simulink model "Simulation"  (R2021b)
settings: Solver=FixedStepAuto  StartTime=0.0  StopTime=30  FixedStep=Ts  RelTol=1e-3
InitFcn:
  | Tf = 200;
  | Ts = 0.01;
  | T = 0:Ts:Tf;
  | rolla = T';
  | omegaa=T';
  | omegax =T';
  | %%
  | 
  | load('A');
  | A = A(2001:2000+length(T),:);
  | rolla(:,2) = A(:,2)-0.0661;
  | omegaa(:,2) = A(:,1);
  | omegax(:,2) = A(:,3);
  | %%
  | l1 =10;
  | initial_vector_error = ones(1,l1)*0.001;
  | initial_vector_error(1) = 0.001;
undefined symbols (not defined in the file or in its folder): X, Y, Z
libraries: nesl_utility x23, sm_lib x15, simulink x3
(part 2 of 2)

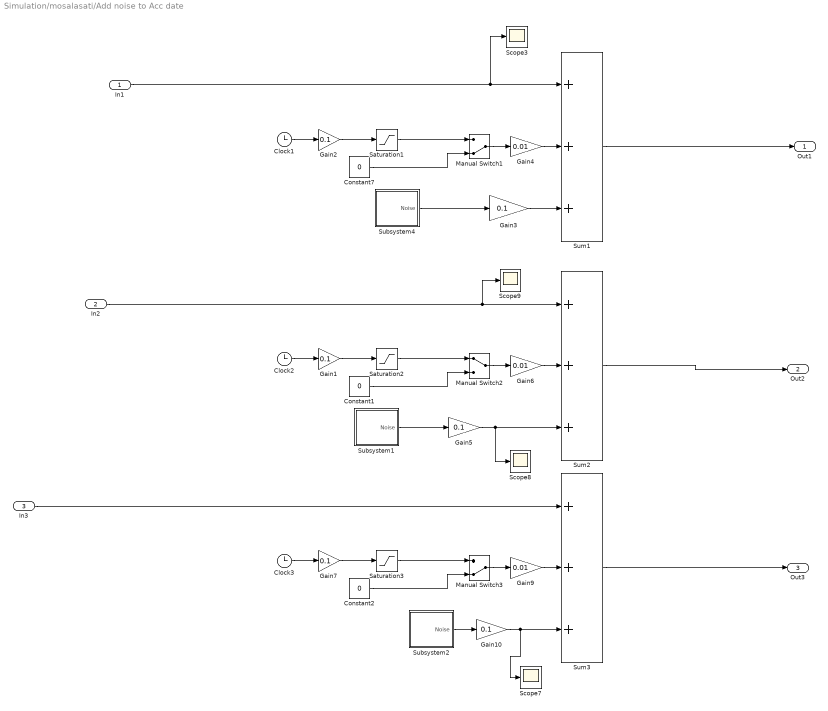
== system Simulation/mosalasati/Add noise to Acc date ==
  In1 : Inport
  In2 : Inport  Port=2
  In3 : Inport  Port=3
  Clock1 : Clock
  Clock2 : Clock
  Clock3 : Clock
  Constant1 : Constant  Value=0
  Constant2 : Constant  Value=0
  Constant7 : Constant  Value=0
  Gain{1..3,5,7,10} (6 alike) : Gain  Gain=0.1
  Gain4 : Gain  Gain=0.01
  Gain6 : Gain  Gain=0.01
  Gain9 : Gain  Gain=0.01
  Manual Switch1 : ManualSwitch  CurrentSetting=0
  Manual Switch2 : ManualSwitch
  Manual Switch3 : ManualSwitch  CurrentSetting=0
  Saturation1 : Saturate  UpperLimit=5
  Saturation2 : Saturate  UpperLimit=5
  Saturation3 : Saturate  UpperLimit=5
  Scope{3,7..9} (4 alike) : Scope
  Subsystem1 : Subsystem
  Subsystem2 : Subsystem
  Subsystem4 : Subsystem
  Sum1 : Sum  Inputs=+++
  Sum2 : Sum  Inputs=+++
  Sum3 : Sum  Inputs=+++
  Out1 : Outport  VectorParamsAs1DForOutWhenUnconnected=off
  Out2 : Outport  Port=2  VectorParamsAs1DForOutWhenUnconnected=off
  Out3 : Outport  Port=3  VectorParamsAs1DForOutWhenUnconnected=off
  wires:
  In2/1 -> Sum2/1, Scope9/1
  Saturation2/1 -> Manual Switch2/1
  Constant1/1 -> Manual Switch2/2
  Gain6/1 -> Sum2/2
  Manual Switch1/1 -> Gain4/1
  Manual Switch2/1 -> Gain6/1
  Sum1/1 -> Out1/1
  Gain7/1 -> Saturation3/1
  Gain2/1 -> Saturation1/1
  Gain3/1 -> Sum1/3
  Constant7/1 -> Manual Switch1/2
  Saturation1/1 -> Manual Switch1/1
  Gain4/1 -> Sum1/2
  Clock1/1 -> Gain2/1
  Gain5/1 -> Scope8/1, Sum2/3
  Clock2/1 -> Gain1/1
  Gain1/1 -> Saturation2/1
  In1/1 -> Scope3/1, Sum1/1
  Subsystem1/1(Noise) -> Gain5/1
  Gain10/1 -> Scope7/1, Sum3/3
  Sum3/1 -> Out3/1
  Saturation3/1 -> Manual Switch3/1
  Subsystem4/1(Noise) -> Gain3/1
  Subsystem2/1(Noise) -> Gain10/1
  Constant2/1 -> Manual Switch3/2
  Clock3/1 -> Gain7/1
  Manual Switch3/1 -> Gain9/1
  Gain9/1 -> Sum3/2
  In3/1 -> Sum3/1
  Sum2/1 -> Out2/1

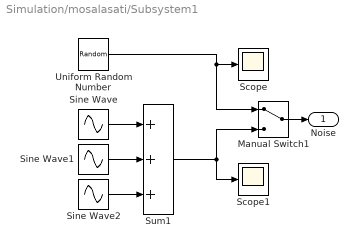
== system Simulation/mosalasati/Subsystem1 ==
  Manual Switch1 : ManualSwitch
  Scope : Scope
  Scope1 : Scope
  Sine Wave : Sin  Amplitude=0.005  Bias=0.001  Frequency=120  Phase=1  SampleTime=0
  Sine Wave1 : Sin  Amplitude=0.02  Frequency=60  Phase=2  SampleTime=0
  Sine Wave2 : Sin  Amplitude=0.04  Frequency=90  Phase=9.54  SampleTime=0
  Sum1 : Sum  Inputs=+++
  Uniform Random Number : UniformRandomNumber  SampleTime=0.1
  Noise : Outport  VectorParamsAs1DForOutWhenUnconnected=off
  wires:
  Uniform Random Number/1 -> Scope/1, Manual Switch1/1
  Sine Wave1/1 -> Sum1/2
  Sum1/1 -> Scope1/1, Manual Switch1/2
  Manual Switch1/1 -> Noise/1
  Sine Wave/1 -> Sum1/1
  Sine Wave2/1 -> Sum1/3

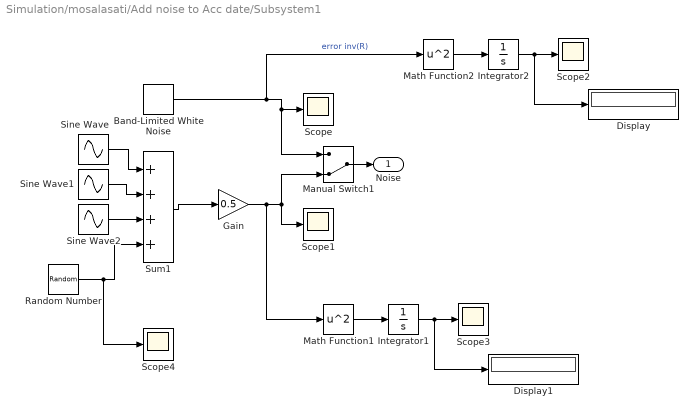
== system Simulation/mosalasati/Add noise to Acc date/Subsystem1 ==
  Band-Limited White Noise : simulink/Sources/Band-Limited White Noise  Cov=0.000004  Ts=0.01  seed=[23341]
  Display : Display
  Display1 : Display
  Gain : Gain  Gain=0.5
  Integrator1 : Integrator
  Integrator2 : Integrator
  Manual Switch1 : ManualSwitch  CurrentSetting=0
  Math Function1 : Math  Operator=square  SignedPower=on  SaturateOnIntegerOverflow=on
  Math Function2 : Math  Operator=square  SignedPower=on  SaturateOnIntegerOverflow=on
  Random Number : RandomNumber  Variance=0.001
  Scope{,1..4} (5 alike) : Scope
  Sine Wave : Sin  Amplitude=0.005  Bias=0.001  Frequency=120  Phase=1  SampleTime=0
  Sine Wave1 : Sin  Amplitude=0.02  Frequency=60  Phase=2  SampleTime=0
  Sine Wave2 : Sin  Amplitude=0.04  Frequency=90  Phase=9.54  SampleTime=0
  Sum1 : Sum  Inputs=++++
  Noise : Outport  VectorParamsAs1DForOutWhenUnconnected=off
  wires:
  Math Function1/1 -> Integrator1/1
  Integrator1/1 -> Display1/1, Scope3/1
  Integrator2/1 -> Scope2/1, Display/1
  Math Function2/1 -> Integrator2/1
  Band-Limited White Noise/1 -> Scope/1, Manual Switch1/1, Math Function2/1  "error inv(R)"
  Gain/1 -> Scope1/1, Manual Switch1/2, Math Function1/1
  Random Number/1 -> Sum1/4, Scope4/1
  Sine Wave1/1 -> Sum1/2
  Sum1/1 -> Gain/1
  Manual Switch1/1 -> Noise/1
  Sine Wave/1 -> Sum1/1
  Sine Wave2/1 -> Sum1/3

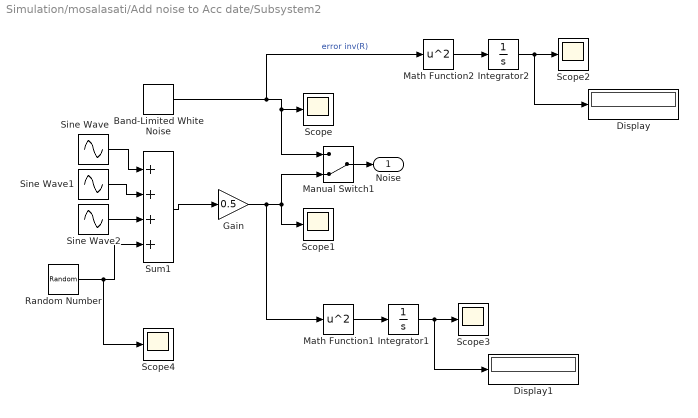
== system Simulation/mosalasati/Add noise to Acc date/Subsystem2 ==
  Band-Limited White Noise : simulink/Sources/Band-Limited White Noise  Cov=0.000004  Ts=0.01  seed=[23341]
  Display : Display
  Display1 : Display
  Gain : Gain  Gain=0.5
  Integrator1 : Integrator
  Integrator2 : Integrator
  Manual Switch1 : ManualSwitch  CurrentSetting=0
  Math Function1 : Math  Operator=square  SignedPower=on  SaturateOnIntegerOverflow=on
  Math Function2 : Math  Operator=square  SignedPower=on  SaturateOnIntegerOverflow=on
  Random Number : RandomNumber  Variance=0.001
  Scope{,1..4} (5 alike) : Scope
  Sine Wave : Sin  Amplitude=0.005  Bias=0.001  Frequency=120  Phase=1  SampleTime=0
  Sine Wave1 : Sin  Amplitude=0.02  Frequency=60  Phase=2  SampleTime=0
  Sine Wave2 : Sin  Amplitude=0.04  Frequency=90  Phase=9.54  SampleTime=0
  Sum1 : Sum  Inputs=++++
  Noise : Outport  VectorParamsAs1DForOutWhenUnconnected=off
  wires:
  Sine Wave2/1 -> Sum1/3
  Sine Wave/1 -> Sum1/1
  Manual Switch1/1 -> Noise/1
  Sum1/1 -> Gain/1
  Sine Wave1/1 -> Sum1/2
  Random Number/1 -> Scope4/1, Sum1/4
  Gain/1 -> Math Function1/1, Manual Switch1/2, Scope1/1
  Band-Limited White Noise/1 -> Math Function2/1, Manual Switch1/1, Scope/1  "error inv(R)"
  Math Function2/1 -> Integrator2/1
  Integrator2/1 -> Display/1, Scope2/1
  Integrator1/1 -> Scope3/1, Display1/1
  Math Function1/1 -> Integrator1/1

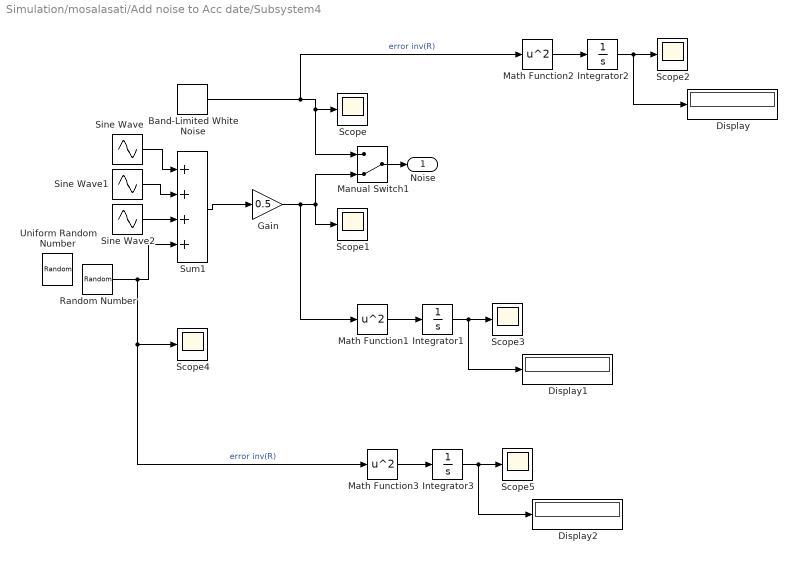
== system Simulation/mosalasati/Add noise to Acc date/Subsystem4 ==
  Band-Limited White Noise : simulink/Sources/Band-Limited White Noise  Cov=0.000004  Ts=0.01  seed=[23341]
  Display : Display
  Display1 : Display
  Display2 : Display
  Gain : Gain  Gain=0.5
  Integrator1 : Integrator
  Integrator2 : Integrator
  Integrator3 : Integrator
  Manual Switch1 : ManualSwitch  CurrentSetting=0
  Math Function1 : Math  Operator=square  SignedPower=on  SaturateOnIntegerOverflow=on
  Math Function2 : Math  Operator=square  SignedPower=on  SaturateOnIntegerOverflow=on
  Math Function3 : Math  Operator=square  SignedPower=on  SaturateOnIntegerOverflow=on
  Random Number : RandomNumber  Variance=0.001
  Scope{,1..5} (6 alike) : Scope
  Sine Wave : Sin  Amplitude=0.005  Bias=0.001  Frequency=120  Phase=1  SampleTime=0
  Sine Wave1 : Sin  Amplitude=0.02  Frequency=60  Phase=2  SampleTime=0
  Sine Wave2 : Sin  Amplitude=0.04  Frequency=90  Phase=9.54  SampleTime=0
  Sum1 : Sum  Inputs=++++
  Uniform Random Number : UniformRandomNumber  SampleTime=0.1
  Noise : Outport  VectorParamsAs1DForOutWhenUnconnected=off
  wires:
  Sine Wave2/1 -> Sum1/3
  Sine Wave/1 -> Sum1/1
  Manual Switch1/1 -> Noise/1
  Sum1/1 -> Gain/1
  Sine Wave1/1 -> Sum1/2
  Gain/1 -> Math Function1/1, Manual Switch1/2, Scope1/1
  Band-Limited White Noise/1 -> Math Function2/1, Manual Switch1/1, Scope/1  "error inv(R)"
  Math Function2/1 -> Integrator2/1
  Integrator2/1 -> Display/1, Scope2/1
  Integrator1/1 -> Scope3/1, Display1/1
  Math Function1/1 -> Integrator1/1
  Integrator3/1 -> Scope5/1, Display2/1
  Math Function3/1 -> Integrator3/1
  Random Number/1 -> Math Function3/1, Scope4/1, Sum1/4  "error inv(R)"

== matlab function Simulation/mosalasati/MATLAB Function1 ==
  data: ax input; ay input; accAngley output; az input
function accAngley = fcn(ax,ay,az)

b = atan2(-1,sqrt(2));
accAngley = (atan2(-ax,sqrt(ay^2+az^2))-b)*180/pi;
end

== matlab function Simulation/Simscape Model/MATLAB Function ==
  data: yaw input; ax output; pitch input; roll input; ay output; az output
function [ax,ay,az] = fcn(yaw,pitch,roll)
    
ay = cos(pitch)*sin(roll);
az = cos(pitch)*cos(roll);
ax = sin(pitch);

== matlab function Simulation/Kalma filter3/K ==
  data: Ts input; uk input; zk input; P_k_plus_a output; P_k_a input; x_had_a input; K_k_a output; x_k_plus_a output; v_k output; Q_hat input; R_hat input; Q_hat_plus output; R_hat_plus output; i_old input; i output; norm_error_old input; norm_error output
function [P_k_plus_a,K_k_a,x_k_plus_a,v_k,Q_hat_plus,R_hat_plus,i,norm_error] = fcn(Ts,uk,zk,P_k_a,x_had_a,Q_hat,R_hat,i_old,norm_error_old)
    %Ts = 0.01;
    F = [1,Ts;0,1];
    G = [Ts;0];
    H = [1,Ts];
    %%
%     Q_hat = Q_k;
%     R_hat = R_k;
    R_hat_2=0.01;
    %% Kalman Filter
    P_k_minus_a = F*P_k_a*transpose(F) + Q_hat;
    x_k_minus_a = F*x_had_a + G*uk;
    K_k_a = P_k_minus_a*transpose(H)*inv(H*P_k_minus_a*transpose(H) + R_hat_2);
    P_k_plus_a = 1*(eye(size(P_k_a))-K_k_a*H)*P_k_minus_a;
    %P_k_plus_a = (eye(size(P_k_a))-K_k_a*H)*P_k_minus_a*transpose((eye(size(P_k_a))-K_k_a*H)) + K_k_a*R_hat*(H);
    x_k_plus_a = x_k_minus_a + K_k_a*(zk - H*x_k_minus_a);
    
    i = i_old+1;
    v_k = zk - H*x_k_plus_a; 
    dk = zk - H*x_k_minus_a;
    norm_error = norm_error_old + v_k^2;

    %  Adaption for Q and R

    
   
    C_hat = norm_error/i;
    Q_hat_plus = K_k_a*C_hat*(K_k_a');
    R_hat_plus = max(C_hat- H*P_k_minus_a*H',0.1);
     
     

end

== matlab function Simulation/Kalma filter/Kalma ==
  data: Ts input; uk input; zk input; P_k_plus output; P_k input; x_had input; K_k output; x_k_plus output; error output
function [P_k_plus,K_k,x_k_plus,error] = fcn(Ts,uk,zk,P_k,x_had)
    %Ts = 0.01;
    F = [1,Ts;0,1];
    G = [Ts;0];
    H = [1,Ts];
    %%
    Q = 0.02*eye(size(F));
    R = 0.07;
    %% Kalman Filter
    P_k_minus = F*P_k*transpose(F) + Q;
    x_k_minus = F*x_had + G*uk;
    K_k = P_k_minus*transpose(H)*inv(H*P_k_minus*transpose(H) + R);
    %zk = H*x_k_minus;
    x_k_plus = x_k_minus + K_k*(zk - H*x_k_minus);
   % P_k_plus = (eye(size(P_k))-K_k*H)*P_k_minus*transpose(eye(size(P_k))-K_k*H) + K_k*R*transpose(K_k);
    P_k_plus = (eye(size(P_k))-K_k*H)*P_k_minus;
    error = zk - H*x_k_minus;
end

== matlab function Simulation/mosalasati/MATLAB Function ==
  data: ay input; accAnglex output; az input; bias input
function accAnglex = fcn(ay,az,bias)

accAnglex = atan2(ay,az)*180/pi;
end

== matlab function Simulation/Kalma filter1/K ==
  data: Ts input; uk input; zk input; P_k_plus_a output; P_k_a input; x_had_a input; K_k_a output; x_k_plus_a output; error output; Q_hat input; R_hat input; Q_hat_plus output; R_hat_plus output; i_old input; i output; norm_error_old input; norm_error output; alpha output; sigmaR output; landa output
function [P_k_plus_a,K_k_a,x_k_plus_a,error,Q_hat_plus,R_hat_plus,i,norm_error,alpha,sigmaR,landa] = fcn(Ts,uk,zk,P_k_a,x_had_a,Q_hat,R_hat,i_old,norm_error_old)
    %Ts = 0.01;
    F = [1,Ts;0,1];
    G = [Ts;0];
    H = [1,Ts];
    rho = 0.5;
    c1 = 0.9;
    c2 = 0.05;
    %%
%     Q_hat = Q_k;
%     R_hat = R_k;
%R_hat=0.5;
    %% Kalman Filter
    P_k_minus_a = F*P_k_a*transpose(F) + Q_hat;
    x_k_minus_a = F*x_had_a + G*uk;
    K_k_a = P_k_minus_a*transpose(H)*inv(H*P_k_minus_a*transpose(H) + R_hat);
    P_k_plus_a = 1*(eye(size(P_k_a))-K_k_a*H)*P_k_minus_a;
    %P_k_plus_a = (eye(size(P_k_a))-K_k_a*H)*P_k_minus_a*transpose((eye(size(P_k_a))-K_k_a*H)) + K_k_a*R_hat*(H);
    x_k_plus_a = x_k_minus_a + K_k_a*(zk - H*x_k_minus_a);
    
    i = i_old+1;
    error = zk - H*x_k_plus_a; 
    norm_error = norm_error_old + error^2;
    landa = norm_error/norm_error_old;
    %  Adaption for Q and R
    deltax=x_k_plus_a - x_k_minus_a;
    deltap=P_k_plus_a - P_k_minus_a;
    
    sigmaQ=rho*deltax*deltax'+(1-rho)*deltap + 0*error^2;
    C_hat = norm_error/i;
    Q_tilda=P_k_plus_a - F*P_k_a*transpose(F)+K_k_a *C_hat*K_k_a';
    alpha=(trace(H*(F*P_k_a*transpose(F) + Q_tilda)*H'))/(trace(H*(F*P_k_a*transpose(F) + Q_hat)*H'));
    if norm(sigmaQ)>=c1
        Q_hat_plus=((alpha))*((sigmaQ/norm(sigmaQ)).*Q_hat);
     else
        Q_hat_plus=Q_hat;
     end
     
     % for R
     dk = zk - H*x_k_minus_a;
     sigmaR=C_hat + H*P_k_plus_a*H';
     gamma=1/sqrt(i+5);
     if norm(sigmaR)>=c2
         R_hat_plus=gamma*(R_hat)+(1-gamma)*sigmaR;
     else
         R_hat_plus=R_hat;
     end
end

== matlab function Simulation/Kalma filter2/kalman FF ==
  data: Ts input; uk input; zk input; P_k_plus_a output; P_k_a input; x_had_a input; K_k_a output; x_k_plus_a output; error output; Q_hat input; R_hat input; Q_hat_plus output; R_hat_plus output; i_old input; i output; norm_error_old input; norm_error output; alpha output; sigmaQ output; landa output; k output; vector_error_old input; vector_error output; temp output
function [P_k_plus_a,K_k_a,x_k_plus_a,error,Q_hat_plus,R_hat_plus,i,norm_error,alpha,sigmaQ,landa,k,vector_error,temp] = fcn(Ts,uk,zk,P_k_a,x_had_a,Q_hat,R_hat,i_old,norm_error_old,vector_error_old)
    %Ts = 0.01;
    F = [1,Ts;0,1];
    G = [Ts;0];
    H = [1,Ts];
    rho = 0.5;
    %%
%     Q_hat = Q_k;
%     R_hat = R_k;

%R_hat=5;
    %% Kalman Filter
    P_k_minus_a = F*P_k_a*transpose(F) + Q_hat;
    x_k_minus_a = F*x_had_a + G*uk;
    K_k_a = P_k_minus_a*transpose(H)*inv(H*P_k_minus_a*transpose(H) +(R_hat));
  
    P_k_plus_a = (1/1)*(eye(size(P_k_a))-K_k_a*H)*P_k_minus_a;
    
    %P_k_plus_a = (eye(size(P_k_a))-K_k_a*H)*P_k_minus_a*transpose((eye(size(P_k_a))-K_k_a*H)) + K_k_a*R_hat*(H);
    x_k_plus_a = x_k_minus_a + K_k_a*(zk - H*x_k_minus_a);
    
    i = i_old+1;
    error = zk - H*x_k_plus_a;
    temp =  error;
    norm_error  = norm_error_old + error^2;
    % ######################### forgetting factor##########################
    k = ((mean(vector_error_old)+10*error^2)/mean(vector_error_old))^1; 
    vector_error = circshift(vector_error_old,1); 
    vector_error(1) = error^2;                         
    norm_error2 = norm_error_old + k*error^2;  
    landa = norm_error2/norm_error_old; 
    P_k_plus_a = landa*P_k_plus_a;     
    % ######################### forgetting factor##########################
    %  Adaption for Q and R
    deltax=x_k_plus_a - x_k_minus_a; 
    deltap=P_k_plus_a - P_k_minus_a; 
    
    sigmaQ=rho*deltax*deltax'+(1-rho)*deltap + 0*error^2; 
    C_hat = norm_error/i;
    Q_tilda=P_k_plus_a - F*P_k_a*transpose(F)+K_k_a *C_hat*K_k_a'; 
    alpha=(trace(H*(F*P_k_a*transpose(F) + Q_tilda)*H'))/(trace(H*(F*P_k_a*transpose(F) + Q_hat)*H')); 
    if norm(sigmaQ)>=0.1
        Q_hat_plus=((alpha))*((sigmaQ/norm(sigmaQ)).*Q_hat);
     else
        Q_hat_plus=Q_hat;
    end
     % for R
     sigmaR=error^2 + H*P_k_plus_a*H';
     gamma=1/sqrt(i+5);
     if norm(sigmaR)>=20
         R_hat_plus=gamma*(R_hat)+(1-gamma)*(1/trace(R_hat))*sigmaR.*R_hat;
     else
         R_hat_plus=R_hat;
     end
    Q_hat_plus = K_k_a*C_hat*(K_k_a');
    R_hat_plus = max(C_hat- H*P_k_minus_a*H',0.1);
     
end
